simulink model "heat_pump_model"  (R2020b)
settings: Solver=VariableStepAuto  StartTime=0.0  StopTime=2000  RelTol=1e-3
undefined symbols (not defined in the file): A1, A2, A3, A4, A5, Cp1, Cp2, Cp3, Cp4, Cp6, Cp7, Cp8, m1, m10, m11, m2, m3, m4, m5, m6, m8, m9, mdot, mdot1, mdot2, mdot3, Pin, T1, T2, T3, T4, Tc, Td, Tgo, Ti, To, U1, U2, U3, U4, U5, U6, U7
settings Model: Creator=Atheesh  LastModifiedBy=Atheesh

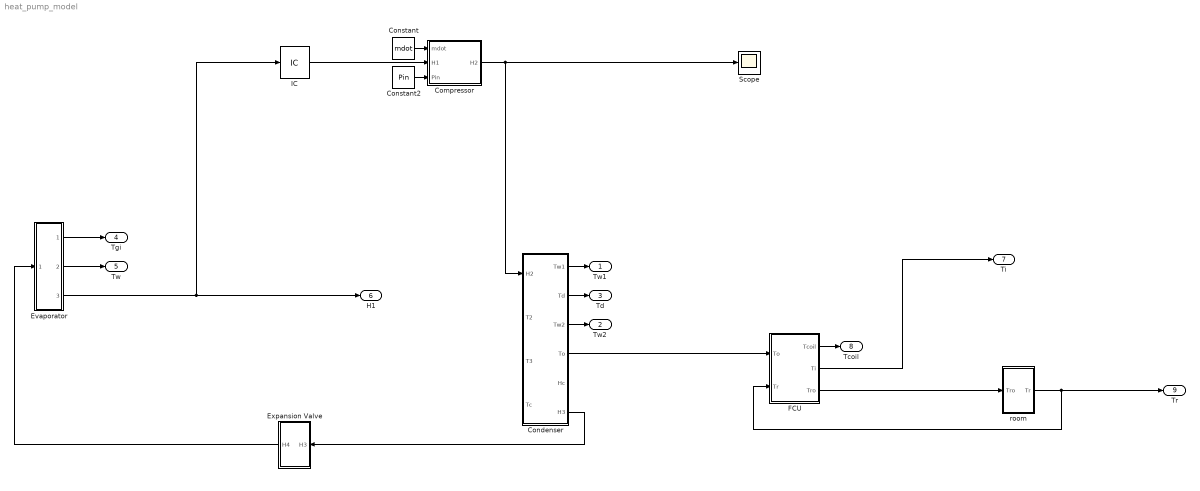
== system heat_pump_model ==
  Compressor : Subsystem
  Condenser : Subsystem
  Constant : Constant  Value=mdot
  Constant2 : Constant  Value=Pin
  Evaporator : Subsystem
  Expansion Valve : Subsystem
  FCU : Subsystem
  IC : InitialCondition
  Scope : Scope
  room : Subsystem
  Tw1 : Outport
  Tw2 : Outport  Port=2
  Td : Outport  Port=3
  Tgi : Outport  Port=4
  Tw : Outport  Port=5
  H1 : Outport  Port=6
  Ti : Outport  Port=7
  Tcoil : Outport  Port=8
  Tr : Outport  Port=9
  wires:
  FCU/2(Ti) -> Ti/1
  FCU/3(Tro) -> room/1(Tro)
  FCU/1(Tcoil) -> Tcoil/1
  Evaporator/1(Out1) -> Tgi/1
  Evaporator/2(Out2) -> Tw/1
  Condenser/4(To) -> FCU/1(To)
  Evaporator/3(Out3) -> IC/1, H1/1
  Constant/1 -> Compressor/1(mdot)
  IC/1 -> Compressor/2(H1)
  Constant2/1 -> Compressor/3(Pin)
  Condenser/3(Tw2) -> Tw2/1
  Condenser/2(Td) -> Td/1
  Condenser/1(Tw1) -> Tw1/1
  room/1(Tr) -> FCU/2(Tr), Tr/1
  Compressor/1(H2) -> Condenser/1(H2), Scope/1
  Condenser/6(H3) -> Expansion Valve/1(H3)
  Expansion Valve/1(H4) -> Evaporator/1(H4)

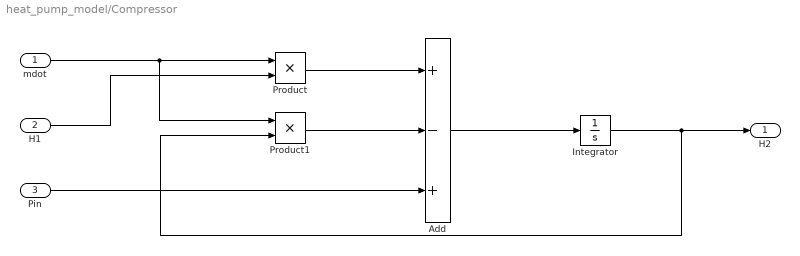
== system heat_pump_model/Compressor ==
  mdot : Inport
  H1 : Inport  Port=2
  Pin : Inport  Port=3
  Add : Sum  Inputs=+-+
  Integrator : Integrator
  Product : Product
  Product1 : Product
  H2 : Outport
  wires:
  Add/1 -> Integrator/1
  mdot/1 -> Product/1, Product1/1
  Integrator/1 -> H2/1, Product1/2
  Pin/1 -> Add/3
  Product/1 -> Add/1
  Product1/1 -> Add/2
  H1/1 -> Product/2

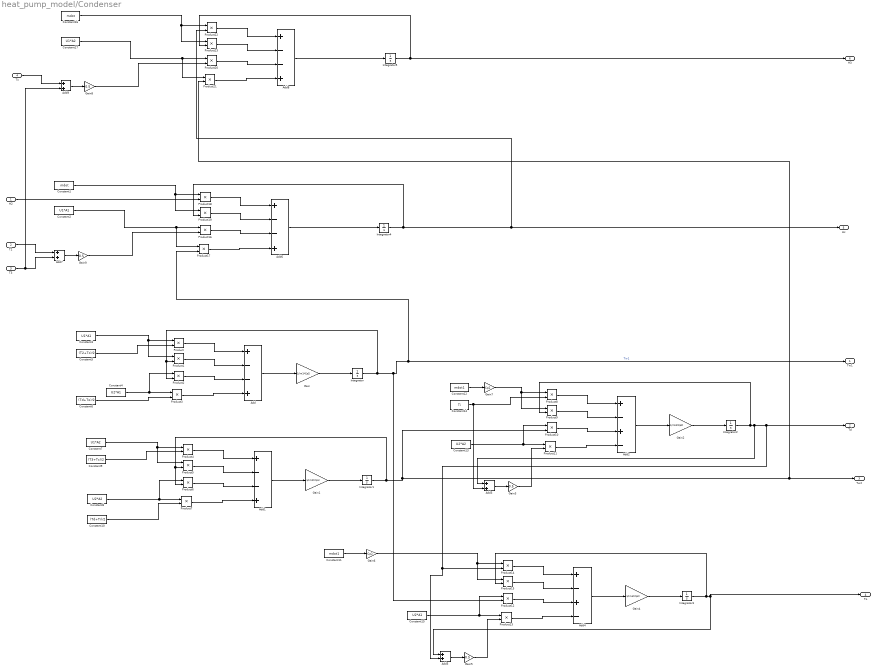
== system heat_pump_model/Condenser ==
  H2 : Inport
  T2 : Inport  Port=2
  T3 : Inport  Port=3
  Tc : Inport  Port=4
  Add{,1,6,8} (4 alike) : Sum  Inputs=+--+
  Add2 : Sum  Inputs=+-+-
  Add{3,5,7,9} (4 alike) : Sum
  Add4 : Sum  Inputs=+-+-
  Constant1 : Constant  Value=mdot
  Constant10 : Constant  Value=(Td+Ti)/2
  Constant11 : Constant  Value=mdot1
  Constant12 : Constant  Value=mdot1
  Constant13 : Constant  Value=U2*A2
  Constant14 : Constant  Value=Ti
  Constant15 : Constant  Value=U2*A1
  Constant16 : Constant  Value=mdot
  Constant17 : Constant  Value=U1*A2
  Constant2 : Constant  Value=U1*A1
  Constant3 : Constant  Value=U1*A1
  Constant4 : Constant  Value=U2*A1
  Constant5 : Constant  Value=(T2+Tc)/2
  Constant6 : Constant  Value=(Td+To)/2
  Constant7 : Constant  Value=U1*A2
  Constant8 : Constant  Value=U2*A2
  Constant9 : Constant  Value=(T3+Tc)/2
  Gain : Gain  Gain=1/(m1*Cp1)
  Gain1 : Gain  Gain=1/(m2*Cp1)
  Gain2 : Gain  Gain=1/(m3*Cp2)
  Gain{3,5,8..9} (4 alike) : Gain  Gain=0.5
  Gain4 : Gain  Gain=1/(m4*Cp2)
  Gain6 : Gain  Gain=Cp2
  Gain7 : Gain  Gain=Cp2
  Integrator{,1..5} (6 alike) : Integrator
  Product{,1..23} (24 alike) : Product
  Tw1 : Outport
  Td : Outport  Port=2
  Tw2 : Outport  Port=3
  To : Outport  Port=4
  Hc : Outport  Port=5
  H3 : Outport  Port=6
  wires:
  Product2/1 -> Add/3
  Product10/1 -> Add2/3
  Constant3/1 -> Product1/1, Product/1
  Constant6/1 -> Product3/2
  Constant13/1 -> Product10/1, Product11/1
  Integrator/1 -> Product2/2, Product1/2, Product17/2, Tw1/1, Product12/2  "Tw1"
  Gain2/1 -> Integrator2/1
  Add1/1 -> Gain1/1
  Product14/1 -> Add4/1
  Constant15/1 -> Product12/1, Product13/1
  Add3/1 -> Gain3/1
  Integrator2/1 -> Product9/2, Add3/1, Td/1, Add5/2, Product14/2
  Gain7/1 -> Product9/1, Product8/1
  Gain/1 -> Integrator/1
  Add2/1 -> Gain2/1
  Gain6/1 -> Product15/1, Product14/1
  Constant5/1 -> Product/2
  Constant7/1 -> Product5/1, Product4/1
  Integrator1/1 -> Product6/2, Product5/2, Product21/2, Tw2/1, Product10/2
  Product11/1 -> Add2/4
  Constant14/1 -> Add3/2, Product8/2
  Constant10/1 -> Product7/2
  Add4/1 -> Gain4/1
  Product8/1 -> Add2/1
  Product3/1 -> Add/4
  Constant4/1 -> Product2/1, Product3/1
  Constant8/1 -> Product6/1, Product7/1
  Product9/1 -> Add2/2
  Constant12/1 -> Gain7/1
  Add/1 -> Gain/1
  Gain4/1 -> Integrator3/1
  Product6/1 -> Add1/3
  Product12/1 -> Add4/3
  Gain1/1 -> Integrator1/1
  Product/1 -> Add/1
  Product1/1 -> Add/2
  Product5/1 -> Add1/2
  Product15/1 -> Add4/2
  Product4/1 -> Add1/1
  Add5/1 -> Gain5/1
  Constant9/1 -> Product4/2
  Product7/1 -> Add1/4
  Gain5/1 -> Product13/2
  Constant11/1 -> Gain6/1
  Integrator3/1 -> Product15/2, To/1, Add5/1
  Product13/1 -> Add4/4
  Gain3/1 -> Product11/2
  Integrator4/1 -> Product22/2, Hc/1, Product19/2
  Product19/1 -> Add6/2
  Product17/1 -> Add6/4
  Product18/1 -> Add6/1
  Add7/1 -> Gain9/1
  Product16/1 -> Add6/3
  Add6/1 -> Integrator4/1
  Constant1/1 -> Product19/1, Product18/1
  Constant2/1 -> Product17/1, Product16/1
  H2/1 -> Product18/2
  Gain9/1 -> Product16/2
  T2/1 -> Add7/1
  T3/1 -> Add9/2, Add7/2
  Constant16/1 -> Product23/1, Product22/1
  Gain8/1 -> Product20/2
  Constant17/1 -> Product21/1, Product20/1
  Product20/1 -> Add8/3
  Add9/1 -> Gain8/1
  Tc/1 -> Add9/1
  Add8/1 -> Integrator5/1
  Product23/1 -> Add8/2
  Product21/1 -> Add8/4
  Integrator5/1 -> H3/1, Product23/2
  Product22/1 -> Add8/1

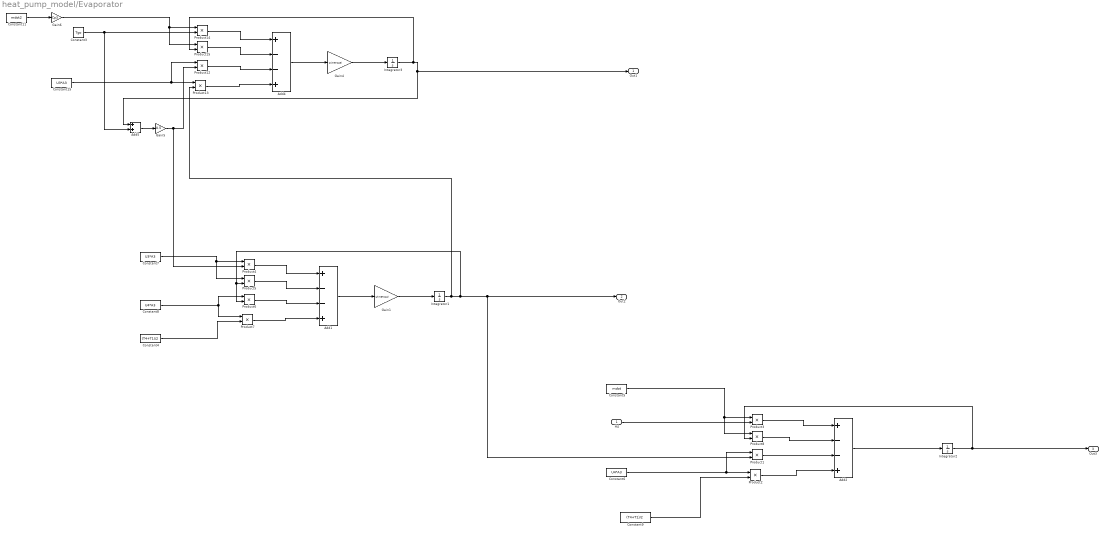
== system heat_pump_model/Evaporator ==
  H4 : Inport
  Add1 : Sum  Inputs=+--+
  Add2 : Sum  Inputs=+--+
  Add4 : Sum  Inputs=+--+
  Add5 : Sum
  Constant11 : Constant  Value=mdot2
  Constant15 : Constant  Value=U3*A3
  Constant3 : Constant  Value=Tgo
  Constant4 : Constant  Value=(T4+T1)/2
  Constant5 : Constant  Value=mdot
  Constant6 : Constant  Value=U4*A3
  Constant7 : Constant  Value=U3*A3
  Constant8 : Constant  Value=U4*A3
  Constant9 : Constant  Value=(T4+T1)/2
  Gain1 : Gain  Gain=1/(m6*Cp4)
  Gain4 : Gain  Gain=1/(m5*Cp3)
  Gain5 : Gain  Gain=0.5
  Gain6 : Gain  Gain=Cp3
  Integrator1 : Integrator
  Integrator2 : Integrator
  Integrator3 : Integrator
  Product{1..8,12..15} (12 alike) : Product
  Out1 : Outport
  Out2 : Outport  Port=2
  Out3 : Outport  Port=3
  wires:
  Gain5/1 -> Product4/2, Product12/2
  Integrator3/1 -> Product15/2, Out1/1, Add5/1
  Constant6/1 -> Product1/1, Product2/1
  Constant9/1 -> Product2/2
  Product13/1 -> Add4/4
  Product5/1 -> Add1/2
  Constant15/1 -> Product12/1, Product13/1
  Product8/1 -> Add2/2
  Integrator1/1 -> Out2/1, Product1/2, Product6/2, Product5/2, Product13/2
  Add4/1 -> Gain4/1
  Constant7/1 -> Product5/1, Product4/1
  Gain6/1 -> Product15/1, Product14/1
  Product14/1 -> Add4/1
  Constant5/1 -> Product8/1, Product3/1
  Product1/1 -> Add2/3
  Gain1/1 -> Integrator1/1
  Add5/1 -> Gain5/1
  Constant8/1 -> Product7/1, Product6/1
  Product15/1 -> Add4/2
  Add2/1 -> Integrator2/1
  Constant11/1 -> Gain6/1
  Product12/1 -> Add4/3
  Product4/1 -> Add1/1
  Gain4/1 -> Integrator3/1
  Add1/1 -> Gain1/1
  Constant3/1 -> Add5/2, Product14/2
  Product2/1 -> Add2/4
  Product7/1 -> Add1/4
  Integrator2/1 -> Out3/1, Product8/2
  Product6/1 -> Add1/3
  Constant4/1 -> Product7/2
  H4/1 -> Product3/2
  Product3/1 -> Add2/1

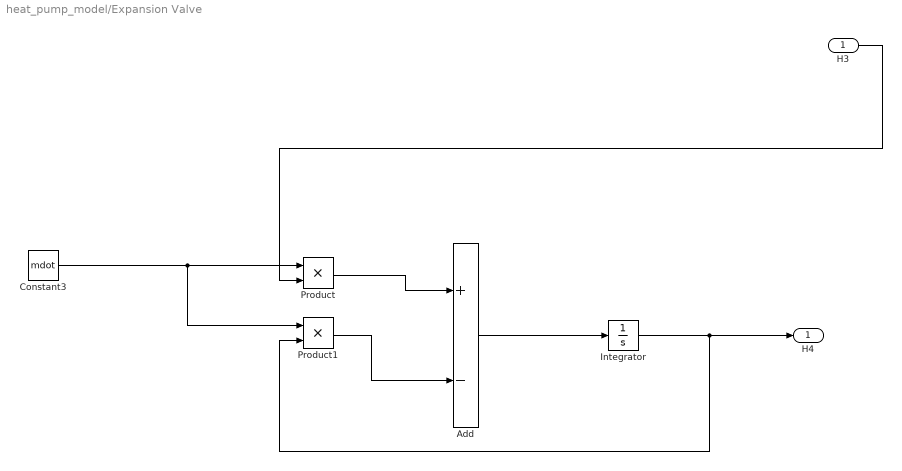
== system heat_pump_model/Expansion Valve ==
  H3 : Inport
  Add : Sum  Inputs=+-
  Constant3 : Constant  Value=mdot
  Integrator : Integrator
  Product : Product
  Product1 : Product
  H4 : Outport
  wires:
  Constant3/1 -> Product/1, Product1/1
  Product1/1 -> Add/2
  Product/1 -> Add/1
  Integrator/1 -> H4/1, Product1/2
  Add/1 -> Integrator/1
  H3/1 -> Product/2

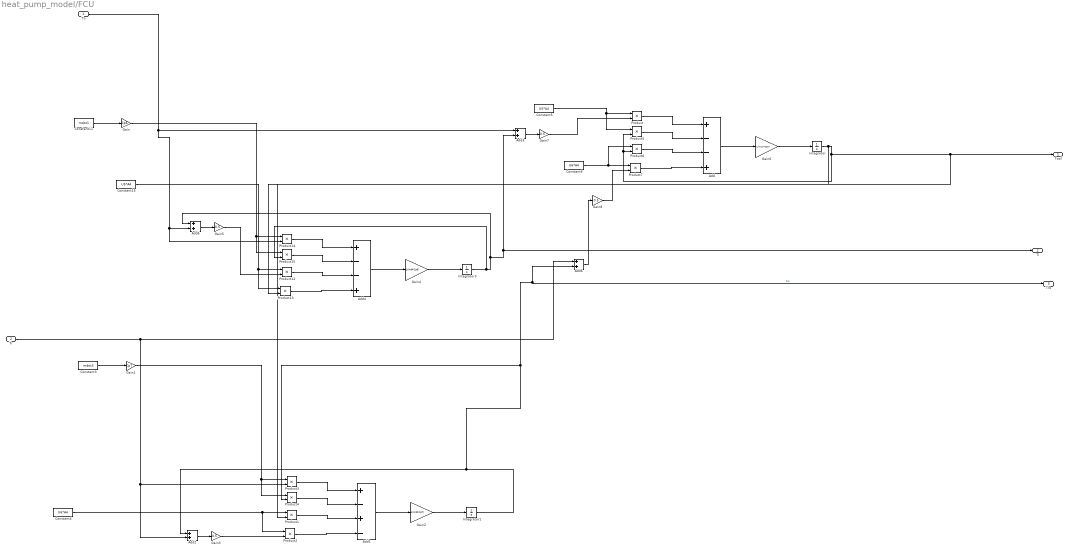
== system heat_pump_model/FCU ==
  To : Inport
  Tr : Inport  Port=2
  Add : Sum  Inputs=+--+
  Add1 : Sum  Inputs=+-+-
  Add{2..3,5..6} (4 alike) : Sum
  Add4 : Sum  Inputs=+--+
  Constant11 : Constant  Value=mdot1
  Constant15 : Constant  Value=U5*A4
  Constant3 : Constant  Value=mdot3
  Constant4 : Constant  Value=U6*A4
  Constant5 : Constant  Value=U5*A4
  Constant6 : Constant  Value=U6*A4
  Gain : Gain  Gain=Cp6
  Gain1 : Gain  Gain=Cp7
  Gain2 : Gain  Gain=1/(m9*Cp7)
  Gain{3,5,7..8} (4 alike) : Gain  Gain=0.5
  Gain4 : Gain  Gain=1/(m8*Cp6)
  Gain6 : Gain  Gain=1/(m10*Cp8)
  Integrator : Integrator
  Integrator1 : Integrator
  Integrator3 : Integrator
  Product{,1..7,12..15} (12 alike) : Product
  Tcoil : Outport
  Ti : Outport  Port=2
  Tro : Outport  Port=3
  wires:
  Gain7/1 -> Product/2
  Constant3/1 -> Gain1/1
  Gain3/1 -> Product2/2
  Integrator1/1 -> Product4/2, Tro/1, Add6/2, Add2/1  "tro"
  Integrator/1 -> Product1/2, Product5/2, Product6/2, Tcoil/1, Product13/2
  Gain8/1 -> Product7/2
  To/1 -> Add3/1, Add5/2, Product14/2
  Product13/1 -> Add4/4
  Constant11/1 -> Gain/1
  Gain4/1 -> Integrator3/1
  Gain1/1 -> Product4/1, Product3/1
  Product15/1 -> Add4/2
  Product14/1 -> Add4/1
  Product3/1 -> Add1/1
  Integrator3/1 -> Product15/2, Add5/1, Ti/1, Add3/2
  Product1/1 -> Add1/3
  Product4/1 -> Add1/2
  Gain6/1 -> Integrator/1
  Product5/1 -> Add/2
  Product6/1 -> Add/3
  Gain2/1 -> Integrator1/1
  Gain5/1 -> Product12/2
  Product/1 -> Add/1
  Gain/1 -> Product15/1, Product14/1
  Add5/1 -> Gain5/1
  Constant4/1 -> Product2/1, Product1/1
  Product12/1 -> Add4/3
  Add1/1 -> Gain2/1
  Constant15/1 -> Product13/1, Product12/1
  Constant6/1 -> Product6/1, Product7/1
  Product2/1 -> Add1/4
  Add2/1 -> Gain3/1
  Product7/1 -> Add/4
  Add4/1 -> Gain4/1
  Tr/1 -> Add2/2, Product3/2, Add6/1
  Add3/1 -> Gain7/1
  Constant5/1 -> Product5/1, Product/1
  Add/1 -> Gain6/1
  Add6/1 -> Gain8/1

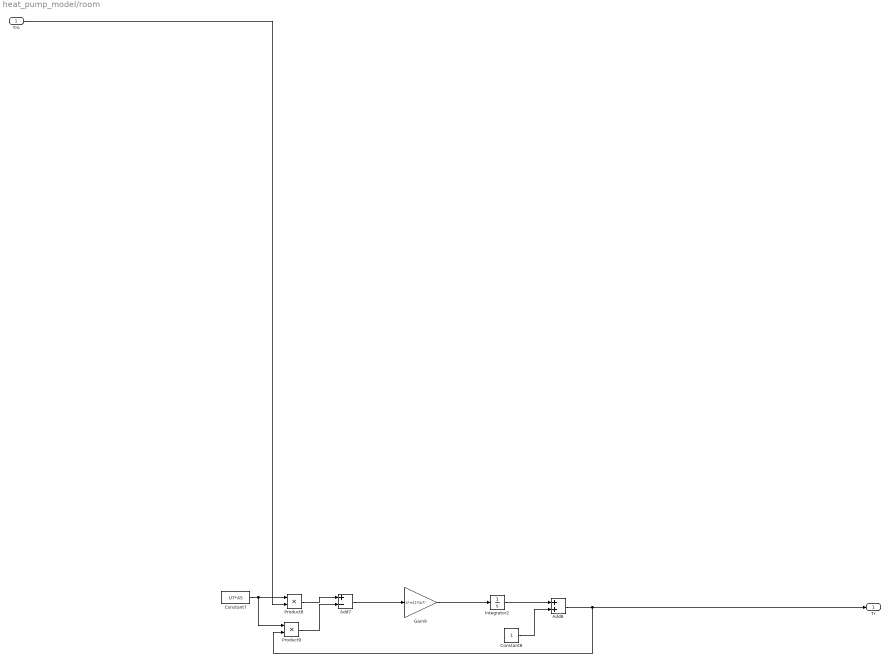
== system heat_pump_model/room ==
  Tro : Inport
  Add7 : Sum  Inputs=+-
  Add8 : Sum
  Constant7 : Constant  Value=U7*A5
  Constant8 : Constant
  Gain9 : Gain  Gain=1/(m11*Cp7)
  Integrator2 : Integrator
  Product8 : Product
  Product9 : Product
  Tr : Outport
  wires:
  Constant8/1 -> Add8/2
  Product9/1 -> Add7/2
  Constant7/1 -> Product9/1, Product8/1
  Add8/1 -> Tr/1, Product9/2
  Add7/1 -> Gain9/1
  Tro/1 -> Product8/2
  Gain9/1 -> Integrator2/1
  Product8/1 -> Add7/1
  Integrator2/1 -> Add8/1
